simulink model "EV_ControlSystem_Architecture_Harness1"  (R2024a)
settings: Solver=FixedStepAuto  StartTime=0.0  StopTime=40  FixedStep=0.1  RelTol=1e-3
undefined symbols (not defined in the file): SOCInit
libraries: SignalEditorBlockLib x2
(part 3 of 3)

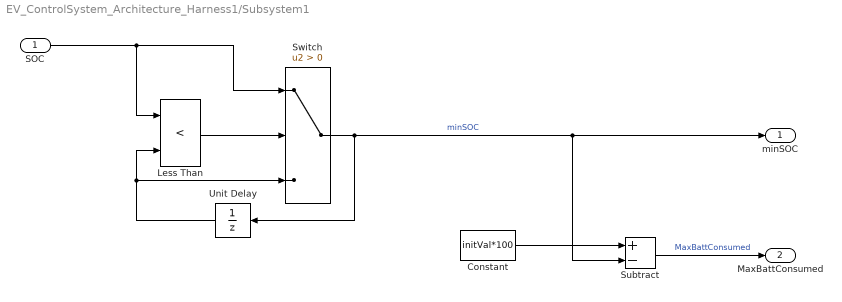
== system EV_ControlSystem_Architecture_Harness1/Subsystem1 ==
  SOC : Inport
  Constant : Constant  Value=initVal*100
  Less Than : RelationalOperator  Operator=<  OutDataTypeStr=boolean  RndMeth=Simplest  InputSameDT=off
  Subtract : Sum  Inputs=+-
  Switch : Switch  Criteria=u2 > Threshold  SaturateOnIntegerOverflow=off  InputSameDT=off
  Unit Delay : UnitDelay  InitialCondition=initVal*100  SampleTime=-1  HasFrameUpgradeWarning=on
  minSOC : Outport
  MaxBattConsumed : Outport  Port=2
  wires:
  Less Than/1 -> Switch/2
  Switch/1 -> Subtract/2, minSOC/1, Unit Delay/1  "minSOC"
  Unit Delay/1 -> Switch/3, Less Than/2
  SOC/1 -> Less Than/1, Switch/1
  Constant/1 -> Subtract/1
  Subtract/1 -> MaxBattConsumed/1  "MaxBattConsumed"

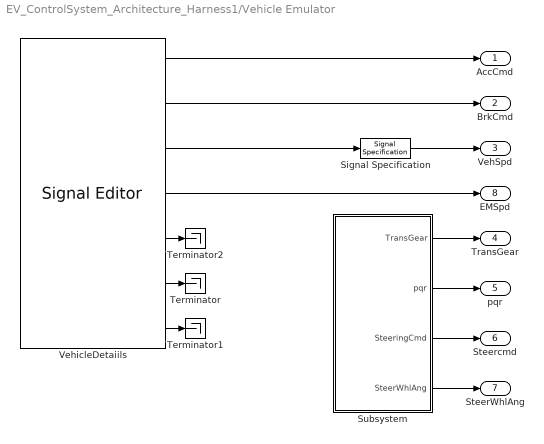
== system EV_ControlSystem_Architecture_Harness1/Vehicle Emulator ==
  Signal Specification : SignalSpecification  Unit=mph
  Subsystem : Subsystem
  Terminator : Terminator
  Terminator1 : Terminator
  Terminator2 : Terminator
  VehicleDetaiils : SignalEditorBlockLib/Signal Editor  FileName=VCUInputs.mat  ActiveScenario=sportMode  ActiveSignal=VehSpd  IsBus=off  OutputBusObjectStr=Bus: BusObject  SampleTime=0  Interpolate=off  ZeroCross=off  OutputAfterFinalValue=Setting to zero  Unit=m/s  PreserveSignalName=on  ApplySigPropsToAllScenarios=on  ApplySigPropsToAllSignals=off
  AccCmd : Outport
  BrkCmd : Outport  Port=2
  VehSpd : Outport  Port=3
  TransGear : Outport  Port=4
  pqr : Outport  Port=5
  Steercmd : Outport  Port=6
  SteerWhlAng : Outport  Port=7
  EMSpd : Outport  Port=8
  wires:
  VehicleDetaiils/1 -> AccCmd/1
  VehicleDetaiils/2 -> BrkCmd/1
  VehicleDetaiils/4 -> EMSpd/1
  VehicleDetaiils/3 -> Signal Specification/1
  Signal Specification/1 -> VehSpd/1
  VehicleDetaiils/6 -> Terminator/1
  VehicleDetaiils/7 -> Terminator1/1
  Subsystem/3(SteeringCmd) -> Steercmd/1
  Subsystem/2(pqr) -> pqr/1
  Subsystem/4(SteerWhlAng) -> SteerWhlAng/1
  VehicleDetaiils/5 -> Terminator2/1
  Subsystem/1(TransGear) -> TransGear/1

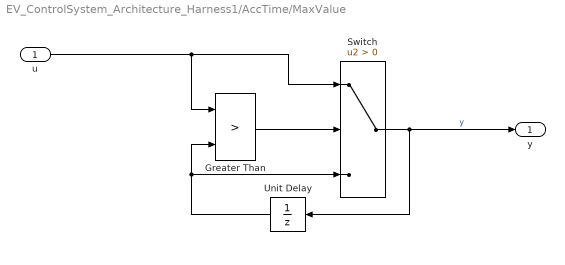
== system EV_ControlSystem_Architecture_Harness1/AccTime/MaxValue ==
  u : Inport
  Greater Than : RelationalOperator  Operator=>  OutDataTypeStr=boolean  RndMeth=Simplest  InputSameDT=off
  Switch : Switch  Criteria=u2 > Threshold  SaturateOnIntegerOverflow=off  InputSameDT=off
  Unit Delay : UnitDelay  SampleTime=-1  HasFrameUpgradeWarning=on
  y : Outport
  wires:
  u/1 -> Switch/1, Greater Than/1
  Unit Delay/1 -> Greater Than/2, Switch/3
  Switch/1 -> Unit Delay/1, y/1  "y"
  Greater Than/1 -> Switch/2

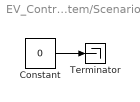
== system EV_ControlSystem_Architecture_Harness1/Subsystem/Scenario ==
  Constant : Constant  Value=0
  Terminator : Terminator
  wires:
  Constant/1 -> Terminator/1

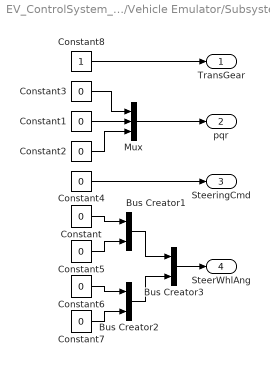
== system EV_ControlSystem_Architecture_Harness1/Vehicle Emulator/Subsystem ==
  Bus Creator1 : BusCreator  Inputs=2
  Bus Creator2 : BusCreator  Inputs=2
  Bus Creator3 : BusCreator  Inputs=2
  Constant{,1..7} (8 alike) : Constant  Value=0
  Constant8 : Constant
  Mux : Mux  Inputs=3
  TransGear : Outport
  pqr : Outport  Port=2
  SteeringCmd : Outport  Port=3
  SteerWhlAng : Outport  Port=4
  wires:
  Constant7/1 -> Bus Creator2/2
  Constant4/1 -> SteeringCmd/1
  Mux/1 -> pqr/1
  Constant1/1 -> Mux/2
  Constant3/1 -> Mux/1
  Bus Creator2/1 -> Bus Creator3/2
  Bus Creator1/1 -> Bus Creator3/1
  Constant/1 -> Bus Creator1/1
  Bus Creator3/1 -> SteerWhlAng/1
  Constant5/1 -> Bus Creator1/2
  Constant6/1 -> Bus Creator2/1
  Constant2/1 -> Mux/3
  Constant8/1 -> TransGear/1

== stateflow chart EV_ControlSystem_Architecture_Harness1/driverInput ==
  state normalMode
    state step_1
      driverMode = 0;
    (default) -> normalMode.step_1
  state sportMode
    state step_1
      driverMode = 1;
    (default) -> sportMode.step_1
  state normalToSportMode
    state step_1
      driverMode = 0;
    state step_2
      driverMode = 1;
    (default) -> normalToSportMode.step_1
    normalToSportMode.step_1 -> step_2 : [
        | after (5.5,sec)
        | ]
  (default) -> normalMode [order 1] : [Active_Scenario_Index == 1]
  (default) -> sportMode [order 2] : [Active_Scenario_Index == 2]
  (default) -> normalToSportMode [order 3] : {assert(Active_Scenario_Index == 3,'The value of Scenario Parameter ''Active_Scenario_Index'' is not valid. Use the index of the scenario to specify it.')}
  data: driverMode output int8; Active_Scenario_Index parameter =2
